simulink model "inlettest"  (R2012b)
settings: Solver=ode45  StartTime=0.0  StopTime=10.0  RelTol=1e-3
settings Model: Creator=tlavelle  LastModifiedBy=tlavelle

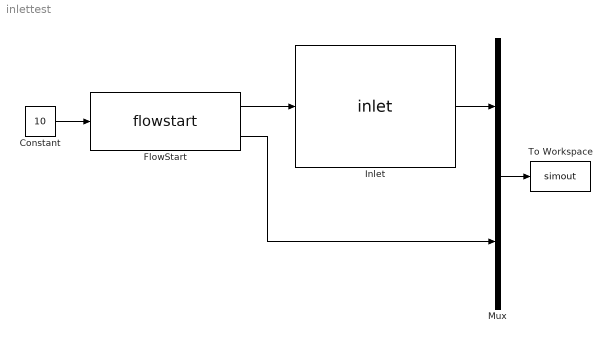
== system inlettest ==
  Constant : Constant  Value=10
  FlowStart : M-S-Function  FunctionName=flowstart  Parameters=Tt,Pt,comp1,comp2,comp3,comp4,comp5,comp6  mask{Tt=500, Pt=15, comp1=1, comp2=0, comp3=0, comp4=0, comp5=0, comp6=0}
      mask prompts: Tt "Exit Temperature"; Pt "Exit Pressure"
      mask Display:
      | color('red'); port_label('input',1,'Flow')
      | color('red'); port_label('output',1,'Flow Out')
  Inlet : M-S-Function  FunctionName=inlet  Parameters=recovery  mask{recovery=.90}
      mask Display:
      | color('red'); port_label('input',1,'Flow In')
      | color('red'); port_label('output',1,'Flow Out')
  Mux : Mux  Inputs=2
  To Workspace : ToWorkspace  VariableName=simout  SampleTime=-1  SaveFormat=Timeseries
  wires:
  Constant/1 -> FlowStart/1
  FlowStart/1 -> Inlet/1
  Inlet/1 -> Mux/1
  Mux/1 -> To Workspace/1
  FlowStart/2 -> Mux/2
